simulink model "FMS_Simu"  (R2022a)
settings: Solver=ode4  StartTime=0.0  StopTime=600  FixedStep=sampletime  RelTol=1e-3
settings Model: Creator=Nguewo  LastModifiedBy=Nguewo
settings SolverCC: AlgebraicLoopSolver=TrustRegion
settings DebuggingCC: UnconnectedInputMsg=warning  UnconnectedOutputMsg=warning  UnconnectedLineMsg=warning  SFMachineParentedDataDiag=warning
settings RTWCC: DLArmComputeVersion=19.05

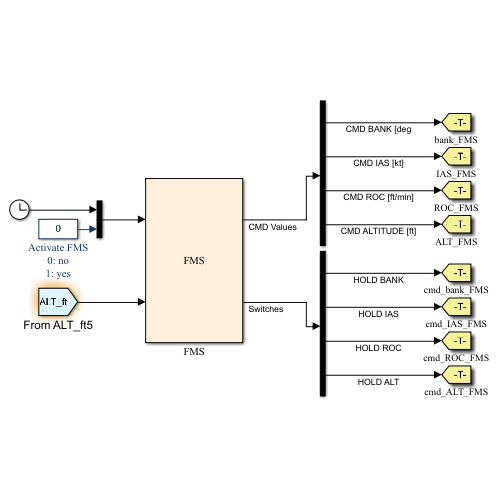
[thumbnail: Simulink's stored preview of the top-level diagram]
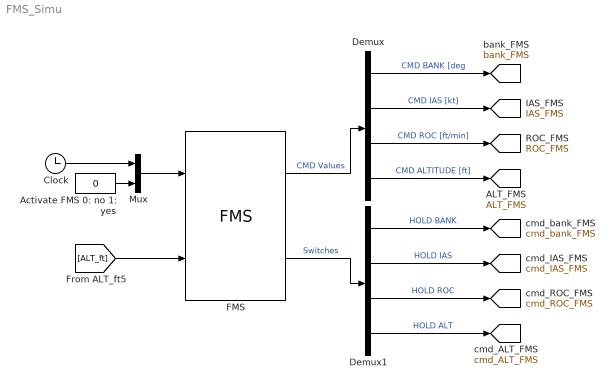
== system FMS_Simu ==
  Activate FMS 0: no 1: yes : Constant  Value=0
  Clock : Clock
  Demux : Demux
  Demux1 : Demux
  FMS : M-S-Function  FunctionName=FMS
  Mux : Mux  Inputs=2
  tag scope: ALT_FMS=global, IAS_FMS=global, ROC_FMS=global, bank_FMS=global, cmd_ALT_FMS=global, cmd_IAS_FMS=global, cmd_ROC_FMS=global, cmd_bank_FMS=global
  wires:
  Clock/1 -> Mux/1
  Activate FMS 0: no 1: yes/1 -> Mux/2
  FMS/1 -> Demux/1  "CMD Values"
  Mux/1 -> FMS/1
  [ALT_ft] -> FMS/2
  FMS/2 -> Demux1/1  "Switches"
  Demux/1 -> [bank_FMS]  "CMD BANK [deg"
  Demux/2 -> [IAS_FMS]  "CMD IAS [kt]"
  Demux/3 -> [ROC_FMS]  "CMD ROC [ft/min]"
  Demux/4 -> [ALT_FMS]  "CMD ALTITUDE [ft]"
  Demux1/1 -> [cmd_bank_FMS]  "HOLD BANK"
  Demux1/2 -> [cmd_IAS_FMS]  "HOLD IAS"
  Demux1/3 -> [cmd_ROC_FMS]  "HOLD ROC"
  Demux1/4 -> [cmd_ALT_FMS]  "HOLD ALT"
